simulink subsystem "clock_and_data_recovery"  (R2022b)
settings: Solver=VariableStepAuto  StartTime=0.0  StopTime=10.0  RelTol=1e-3
settings Model: Creator=Ali-Laptop  LastModifiedBy=Ali-Laptop

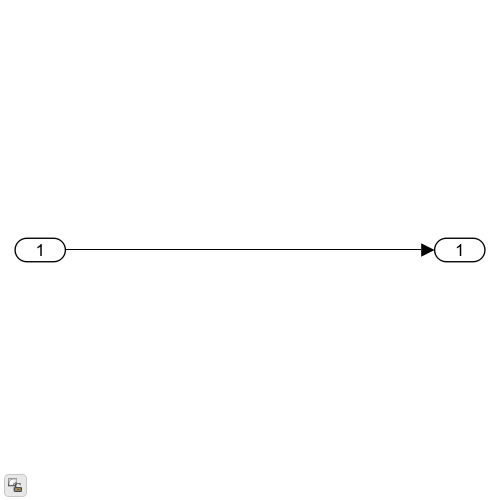
[thumbnail: Simulink's stored preview of the top-level diagram]
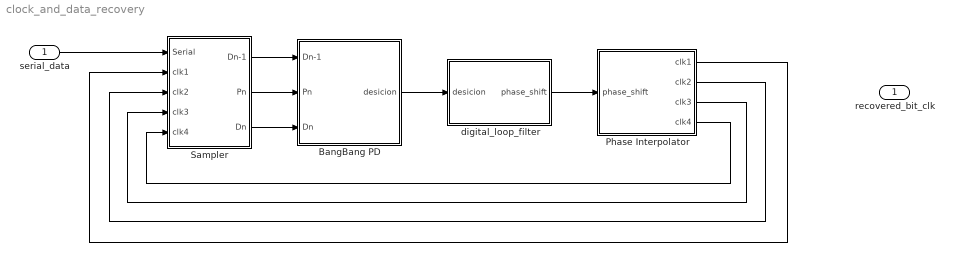
== system clock_and_data_recovery ==
  serial_data : Inport
  BangBang PD : Subsystem
  Phase Interpolator : Subsystem
  Sampler : Subsystem
  digital_loop_filter : Subsystem
  recovered_bit_clk : Outport
  wires:
  BangBang PD/1(desicion) -> digital_loop_filter/1(desicion)
  Sampler/2(Pn) -> BangBang PD/2(Pn)
  Sampler/1(Dn-1) -> BangBang PD/1(Dn-1)
  Sampler/3(Dn) -> BangBang PD/3(Dn)
  digital_loop_filter/1(phase_shift) -> Phase Interpolator/1(phase_shift)
  Phase Interpolator/1(clk1) -> Sampler/2(clk1)
  Phase Interpolator/2(clk2) -> Sampler/3(clk2)
  Phase Interpolator/3(clk3) -> Sampler/4(clk3)
  Phase Interpolator/4(clk4) -> Sampler/5(clk4)
  serial_data/1 -> Sampler/1(Serial)

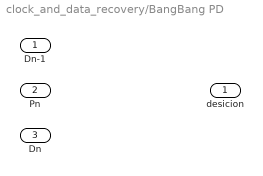
== system clock_and_data_recovery/BangBang PD ==
  Dn-1 : Inport
  Pn : Inport  Port=2
  Dn : Inport  Port=3
  desicion : Outport

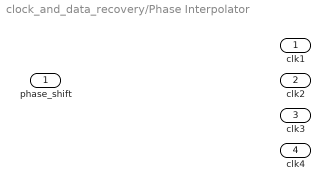
== system clock_and_data_recovery/Phase Interpolator ==
  phase_shift : Inport
  clk1 : Outport
  clk2 : Outport  Port=2
  clk3 : Outport  Port=3
  clk4 : Outport  Port=4

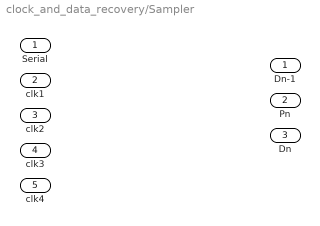
== system clock_and_data_recovery/Sampler ==
  Serial : Inport
  clk1 : Inport  Port=2
  clk2 : Inport  Port=3
  clk3 : Inport  Port=4
  clk4 : Inport  Port=5
  Dn-1 : Outport
  Pn : Outport  Port=2
  Dn : Outport  Port=3

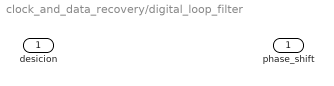
== system clock_and_data_recovery/digital_loop_filter ==
  desicion : Inport
  phase_shift : Outport
